simulink model "slexPowerWindowExample"  (R2014b)
settings: Solver=ode23  StartTime=0  StopTime=10  RelTol=1e-3
PreLoadFcn:
  | if ~exist('CV', 'var') & exist('slexPowerWindowContinuous','file')
  |    slexPowerWindowContinuous
  | end
libraries: slexPowerWindowSALib x8, slrtlib x2, slexPowerWindowDSPLib x2, slexPowerWindowPHYSLib x2, powerlib x1, vrlib x1
CloseFcn:
  | if exist('slexPowerWindowCloseFcn','file')
  |   slexPowerWindowCloseFcn
  | end
Description:
  | Main Power Window Model
settings Model: ModifiedByFormat=The MathWorks Inc.  Creator=The MathWorks Inc.  LastModifiedBy=The MathWorks Inc.
settings SolverCC: InsertRTBMode=Always
settings DataIOCC: SaveFormat=StructureWithTime  InspectSignalLogs=on  SignalLoggingName=sigsOut
settings OptimizationCC: ExpressionDepthLimit=2147483647
settings DebuggingCC: ArrayBoundsChecking=warning  UnderspecifiedInitializationDetection=Classic  MergeDetectMultiDrivingBlocksExec=none  SolverPrmCheckMsg=none  SigSpecEnsureSampleTimeMsg=none  ParameterPrecisionLossMsg=none  StateNameClashWarn=warning
settings ModelReferenceCC: ModelReferencePassRootInputsByReference=off
settings SimMechanicsCC: WarnOnRedundantConstraints=off

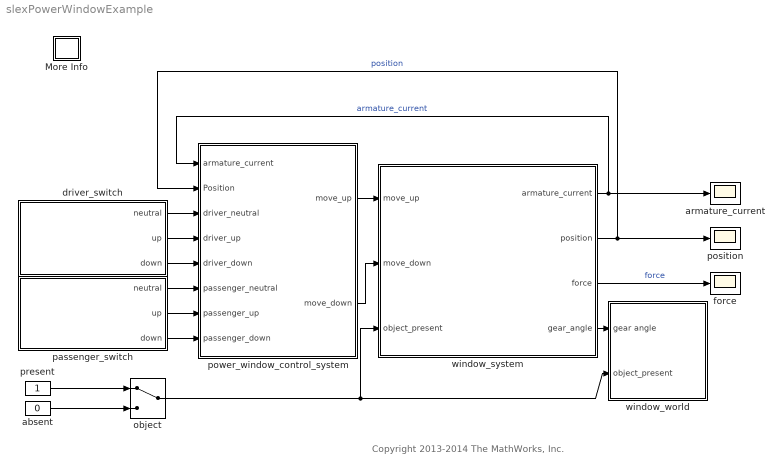
== system slexPowerWindowExample ==
  note: Copyright 2013-2014 The MathWorks, Inc.
  More Info : Subsystem
      settings: OpenFcn=showdemo('slexPowerWindowScript')
      mask Display: disp('?')
  absent : Constant  Value=0  OutDataTypeStr=boolean
  armature_current : Scope
      settings: YMin=-15  YMax=15  SaveName=ScopeData2
  driver_switch : Subsystem  Variant=on
  force : Scope
      settings: YMin=-175  YMax=75  SaveName=ScopeData4
  object : ManualSwitch
  passenger_switch : Subsystem  Variant=on
  position : Scope
      settings: TimeRange=10  YMin=-0.5  YMax=0.5
  power_window_control_system : Subsystem
  present : Constant  OutDataTypeStr=boolean
  window_system : Subsystem  Variant=on
  window_world : Subsystem  LoadFcn=|  Variant=on
      | if license('test','virtual_reality_toolbox') & exist('slexPowerWindowMechWindow.wrl','file')
      |      SL3DBlock = [gcs '/window_world/Simulink_3D_Animation View/VR Sink'];
      |      vrmfunc('FnOpen', get_param(SL3DBlock,'handle'));
      | end
  wires:
  passenger_switch/1(neutral) -> power_window_control_system/6(passenger_neutral)
  passenger_switch/2(up) -> power_window_control_system/7(passenger_up)
  passenger_switch/3(down) -> power_window_control_system/8(passenger_down)
  driver_switch/3(down) -> power_window_control_system/5(driver_down)
  driver_switch/2(up) -> power_window_control_system/4(driver_up)
  driver_switch/1(neutral) -> power_window_control_system/3(driver_neutral)
  power_window_control_system/1(move_up) -> window_system/1(move_up)
  power_window_control_system/2(move_down) -> window_system/2(move_down)
  window_system/1(armature_current) -> power_window_control_system/1(armature_current), armature_current/1  "armature_current"
  window_system/4(gear_angle) -> window_world/1(gear angle)
  window_system/3(force) -> force/1  "force"
  present/1 -> object/1
  absent/1 -> object/2
  window_system/2(position) -> power_window_control_system/2(Position), position/1  "position"
  object/1 -> window_system/3(object_present), window_world/2(object_present)

== system slexPowerWindowExample/More Info ==

== system slexPowerWindowExample/driver_switch ==
  Communication Protocol : Subsystem  VariantControl=V5
  Normal : slexPowerWindowSALib/switch  VariantControl=V1234
  neutral : Outport
  up : Outport  Port=2
  down : Outport  Port=3

== system slexPowerWindowExample/passenger_switch ==
  Communication Protocol : Subsystem  VariantControl=V5
  Normal : slexPowerWindowSALib/switch  VariantControl=V1234
  neutral : Outport
  up : Outport  Port=2
  down : Outport  Port=3

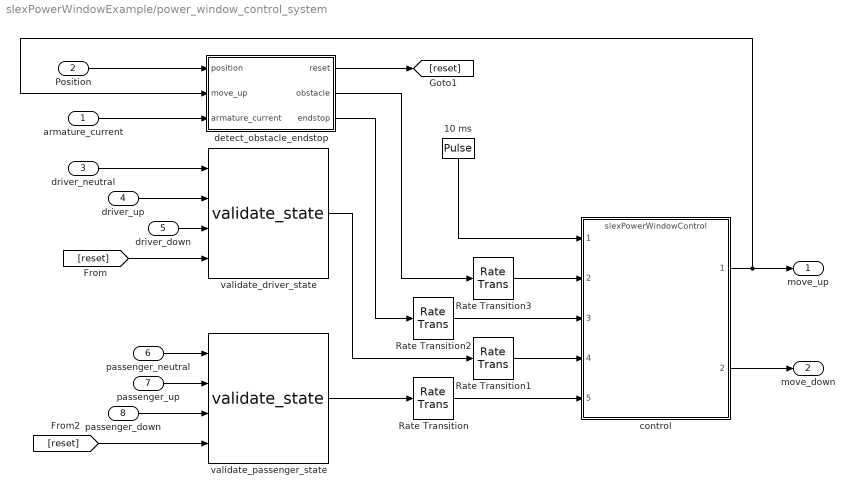
== system slexPowerWindowExample/power_window_control_system ==
  armature_current : Inport
  Position : Inport  Port=2
  driver_neutral : Inport  Port=3
  driver_up : Inport  Port=4
  driver_down : Inport  Port=5
  passenger_neutral : Inport  Port=6
  passenger_up : Inport  Port=7
  passenger_down : Inport  Port=8
  10 ms : DiscretePulseGenerator  SampleTime=10e-3
  Rate Transition{,1..3} (4 alike) : RateTransition
  "control " : ModelReference  ModelNameDialog=slexPowerWindowControl.slx  SimulationMode=Normal  ModelReferenceVersion=1.83  CopyOfModelName=slexPowerWindowControl.slx  DefaultDataLogging=on
  detect_obstacle_endstop : Subsystem  Variant=on
  validate_driver_state : slexPowerWindowSALib/validate_state
  validate_passenger_state : slexPowerWindowSALib/validate_state
  move_up : Outport
  move_down : Outport  Port=2
  wires:
  [reset] -> validate_driver_state/4
  driver_neutral/1 -> validate_driver_state/1
  driver_up/1 -> validate_driver_state/2
  driver_down/1 -> validate_driver_state/3
  detect_obstacle_endstop/1(reset) -> [reset]
  armature_current/1 -> detect_obstacle_endstop/3(armature_current)
  Position/1 -> detect_obstacle_endstop/1(position)
  "control "/1 -> move_up/1, detect_obstacle_endstop/2(move_up)
  "control "/2 -> move_down/1
  passenger_up/1 -> validate_passenger_state/2
  passenger_down/1 -> validate_passenger_state/3
  [reset] -> validate_passenger_state/4
  passenger_neutral/1 -> validate_passenger_state/1
  10 ms/1 -> "control "/1
  validate_passenger_state/1 -> Rate Transition/1
  validate_driver_state/1 -> Rate Transition1/1
  detect_obstacle_endstop/3(endstop) -> Rate Transition2/1
  detect_obstacle_endstop/2(obstacle) -> Rate Transition3/1
  Rate Transition/1 -> "control "/5
  Rate Transition1/1 -> "control "/4
  Rate Transition2/1 -> "control "/3
  Rate Transition3/1 -> "control "/2

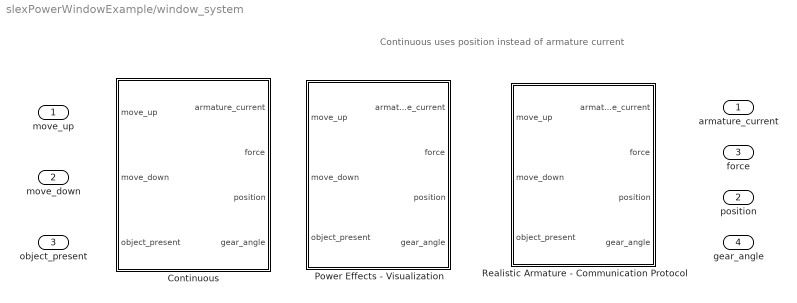
== system slexPowerWindowExample/window_system ==
  note: Continuous uses position instead of armature current
  move_up : Inport
  move_down : Inport  Port=2
  object_present : Inport  Port=3
  Continuous : Subsystem  VariantControl=V1
  Power Effects - Visualization : Subsystem  VariantControl=V23
  Realistic Armature - Communication Protocol : Subsystem  VariantControl=V45
  armature_current : Outport
  position : Outport  Port=2
  force : Outport  Port=3
  gear_angle : Outport  Port=4

== system slexPowerWindowExample/window_world ==
  gear angle : Inport
  object_present : Inport  Port=2
  No_View : Subsystem  VariantControl=V0
  Simulink_3D_Animation View : Subsystem  VariantControl=V12345

== system slexPowerWindowExample/driver_switch/Communication Protocol ==
  driver bit-unpacking1 : slrtlib/CAN/Utilities/CAN bit-unpacking   bitpatterns={ [0:0] [1:1] [2:2] }  dtypes={ 'boolean' 'boolean' 'boolean' }
  driver window control switch : slexPowerWindowDSPLib/driver window control switch
  neutral : Outport
  up : Outport  Port=2
  down : Outport  Port=3
  wires:
  driver window control switch/1 -> driver bit-unpacking1/1
  driver bit-unpacking1/3 -> down/1
  driver bit-unpacking1/1 -> neutral/1
  driver bit-unpacking1/2 -> up/1

== system slexPowerWindowExample/passenger_switch/Communication Protocol ==
  passenger bit-unpacking : slrtlib/CAN/Utilities/CAN bit-unpacking   bitpatterns={ [0:0] [1:1] [2:2] }  dtypes={ 'boolean' 'boolean' 'boolean' }
  passenger window control switch : slexPowerWindowDSPLib/passenger window control switch
  neutral : Outport
  up : Outport  Port=2
  down : Outport  Port=3
  wires:
  passenger bit-unpacking/2 -> up/1
  passenger bit-unpacking/1 -> neutral/1
  passenger bit-unpacking/3 -> down/1
  passenger window control switch/1 -> passenger bit-unpacking/1

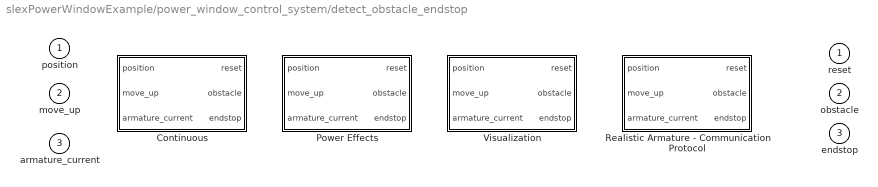
== system slexPowerWindowExample/power_window_control_system/detect_obstacle_endstop ==
  position : Inport
  move_up : Inport  Port=2
  armature_current : Inport  Port=3
  Continuous : Subsystem  VariantControl=V1
  Power Effects : Subsystem  VariantControl=V2
  Realistic Armature - Communication Protocol : Subsystem  VariantControl=V45
  Visualization : Subsystem  VariantControl=V3
  reset : Outport
  obstacle : Outport  Port=2
  endstop : Outport  Port=3

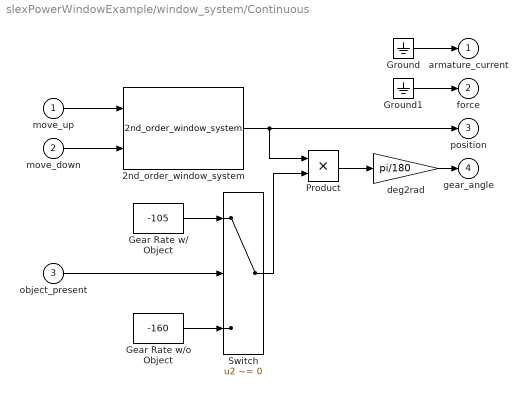
== system slexPowerWindowExample/window_system/Continuous ==
  move_up : Inport
  move_down : Inport  Port=2
  object_present : Inport  Port=3
  2nd_order_window_system : slexPowerWindowSALib/2nd_order_window_system
  Gear Rate w/ Object : Constant  Value=-105
      settings: AttributesFormatString=Units: deg/m
  Gear Rate w/o Object : Constant  Value=-160
      settings: AttributesFormatString=Units: deg/m
  Ground : Ground
  Ground1 : Ground
  Product : Product
  Switch : Switch  Criteria=u2 ~= 0
  deg2rad : Gain  Gain=pi/180
  armature_current : Outport
  force : Outport  Port=2
  position : Outport  Port=3
  gear_angle : Outport  Port=4
  wires:
  move_up/1 -> 2nd_order_window_system/1
  move_down/1 -> 2nd_order_window_system/2
  2nd_order_window_system/1 -> Product/1, position/1
  Ground/1 -> armature_current/1
  Ground1/1 -> force/1
  deg2rad/1 -> gear_angle/1
  object_present/1 -> Switch/2
  Product/1 -> deg2rad/1
  Switch/1 -> Product/2
  Gear Rate w/ Object/1 -> Switch/1
  Gear Rate w/o Object/1 -> Switch/3

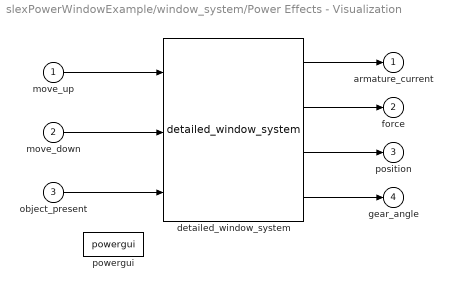
== system slexPowerWindowExample/window_system/Power Effects - Visualization ==
  move_up : Inport
  move_down : Inport  Port=2
  object_present : Inport  Port=3
  detailed_window_system : slexPowerWindowPHYSLib/detailed_window_system
  powergui : powerlib/powergui  SimulationMode=Continuous  SolverType=Tustin  SampleTime=50e-6  frequency=60  SPID=off  DisableSnubberDevices=off  DisableRonSwitches=off  DisableVfSwitches=off  SwTol=0  Interpol=off  DisplayEquations=off  Ts=0  methode=off  frequencyindice=0  Pbase=100e6  ErrMax=1e-4  Iterations=50  UnitsV=kV  UnitsW=MW  FunctionMessages=on  echomessages=off  HookPort=off  EnableUseOfTLC=off  x0status=blocks  RestoreLinks=warning  ResistiveCurrentMeasurement=off  Frange=[0:2:500]  Ylog=off  Xlog=on  ShowGrid=off  save=off  variable=ZData  structure=0  ZoomFFT=on  StartTime=0.0  cycles=1  DisplayStyle=1  fundamental=60  FreqAxis=off  MaxFrequency=1000  frequencyindicesteady=1  RmsSteady=1  display=off
  armature_current : Outport
  force : Outport  Port=2
  position : Outport  Port=3
  gear_angle : Outport  Port=4
  wires:
  detailed_window_system/1 -> armature_current/1
  detailed_window_system/2 -> force/1
  detailed_window_system/3 -> position/1
  detailed_window_system/4 -> gear_angle/1
  move_down/1 -> detailed_window_system/2
  move_up/1 -> detailed_window_system/1
  object_present/1 -> detailed_window_system/3

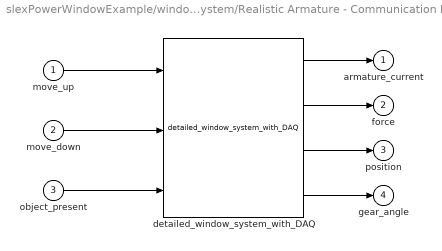
== system slexPowerWindowExample/window_system/Realistic Armature - Communication Protocol ==
  move_up : Inport
  move_down : Inport  Port=2
  object_present : Inport  Port=3
  detailed_window_system_with_DAQ : slexPowerWindowPHYSLib/detailed_window_system_with_DAQ  VariantControl=Variant3
  armature_current : Outport
  force : Outport  Port=2
  position : Outport  Port=3
  gear_angle : Outport  Port=4
  wires:
  detailed_window_system_with_DAQ/1 -> armature_current/1
  detailed_window_system_with_DAQ/2 -> force/1
  detailed_window_system_with_DAQ/3 -> position/1
  detailed_window_system_with_DAQ/4 -> gear_angle/1
  move_down/1 -> detailed_window_system_with_DAQ/2
  move_up/1 -> detailed_window_system_with_DAQ/1
  object_present/1 -> detailed_window_system_with_DAQ/3

== system slexPowerWindowExample/window_world/No_View ==
  gear angle : Inport
  object_present : Inport  Port=2
  Terminator : Terminator
  Terminator1 : Terminator
  wires:
  object_present/1 -> Terminator/1
  gear angle/1 -> Terminator1/1

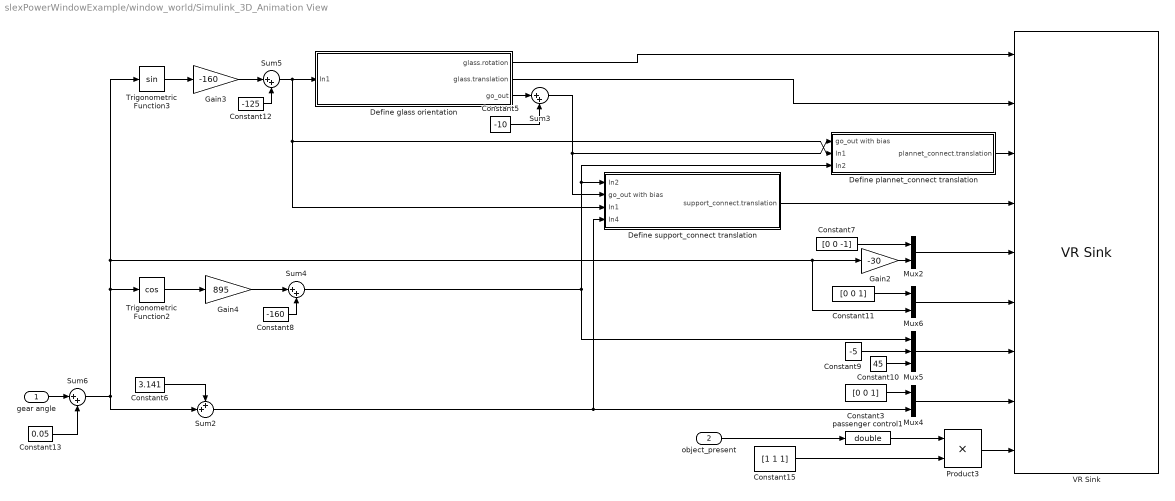
== system slexPowerWindowExample/window_world/Simulink_3D_Animation View ==
  gear angle : Inport
  object_present : Inport  Port=2
  Constant10 : Constant  Value=45
  Constant11 : Constant  Value=[0 0 1]
  Constant12 : Constant  Value=-125
  Constant13 : Constant  Value=0.05
  Constant15 : Constant  Value=[1 1 1]
  Constant3 : Constant  Value=[0 0 1]
  Constant5 : Constant  Value=-10
  Constant6 : Constant  Value=3.141
  Constant7 : Constant  Value=[0 0 -1]
  Constant8 : Constant  Value=-160
  Constant9 : Constant  Value=-5
  Define glass orientation : Subsystem
  Define plannet_connect translation : Subsystem
  Define support_connect translation : Subsystem
  Gain2 : Gain  Gain=-30  SaturateOnIntegerOverflow=on  OutDataTypeStr=Inherit: Same as input  ParamDataTypeStr=Inherit: Same as input
  Gain3 : Gain  Gain=-160  SaturateOnIntegerOverflow=on  OutDataTypeStr=Inherit: Same as input  ParamDataTypeStr=Inherit: Same as input
  Gain4 : Gain  Gain=895  SaturateOnIntegerOverflow=on  OutDataTypeStr=Inherit: Same as input  ParamDataTypeStr=Inherit: Same as input
  Mux2 : Mux  Inputs=2
  Mux4 : Mux  Inputs=2
  Mux5 : Mux  Inputs=3
  Mux6 : Mux  Inputs=2
  Product3 : Product  SaturateOnIntegerOverflow=on  InputSameDT=on  OutDataTypeStr=Inherit: Same as first input
  Sum2 : Sum  Inputs=++|  SaturateOnIntegerOverflow=on  InputSameDT=on  OutDataTypeStr=Inherit: Same as first input
  Sum{3..6} (4 alike) : Sum  Inputs=|++  SaturateOnIntegerOverflow=on  InputSameDT=on  OutDataTypeStr=Inherit: Same as first input
  Trigonometric Function2 : Trigonometry  Operator=cos
  Trigonometric Function3 : Trigonometry
  VR Sink : vrlib/VR Sink  InstantiateOnLoad=on  SampleTime=0.1  ViewEnable=on  RemoteChange=off  RemoteView=on  FieldsWritten=glass.rotation.4.1.1.double#glass.translation.3.1.1.double#plannet_connect.translation.3.1.1.double#support_connect.translation.3.1.1.double#worm.rotation.4.1.1.double#planetROT.rotation.4.1.1.double#support.translation.3.1.1.double#supportROT.rotation.4.1.1.double#balloon.scale.3.1.1.double  WorldFileName=slexPowerWindowMechWindow.wrl  WorldDescription=VR Power Window Model  AutoView=off  VideoDimensions=[]  AllowVariableSize=off  FigureProperties="{'Position', 'Name', 'Viewpoint', 'CameraBound', 'CameraDirection', 'CameraPosition', 'CameraUpVector', 'ZoomFactor', 'Antialiasing', 'Headlight', 'Lighting', 'NavPanel', 'StatusBar', 'ToolBar', 'Textures', 'Transparency', 'Triad', 'Wireframe', 'NavZones', 'NavMode', 'NavSpeed', 'CaptureFileFormat', 'CaptureFileName', 'Record2DCompressMethod', 'Record2DCompressQuality', 'Record2D', 'Record2DFileName', 'Record2DFPS'; [1.0000000000000000e+00   8.9000000000000000e+01   5.8400000000000000e+02   3.8400000000000000e+02], 'VR Power Window Model', 'Main View', 'on', [0.0000000000000000e+00   0.0000000000000000e+00  -1.0000000000000000e+00], [0.0000000000000000e+00   0.0000000000000000e+00   0.0000000000000000e+00], [0.0000000000000000e+00   1.0000000000000000e+00   0.0000000000000000e+00], [1.0000000000000000e+00], 'on', 'on', 'on', 'halfbar', 'on', 'on', 'on', 'on', 'none', 'off', 'off', 'examine', 'normal', 'tif', '%f_anim_%n.tif', 'auto', [7.5000000000000000e+01], 'off', '%f_anim_%n.avi', [1.5000000000000000e+01]}"
  passenger control1 : DataTypeConversion  OutDataTypeStr=double  SaturateOnIntegerOverflow=on  RndMeth=Zero
  wires:
  Mux2/1 -> VR Sink/5
  Mux6/1 -> VR Sink/6
  Mux5/1 -> VR Sink/7
  Define support_connect translation/1(support_connect.translation) -> VR Sink/4
  Product3/1 -> VR Sink/9
  Constant5/1 -> Sum3/2
  Constant7/1 -> Mux2/1
  Gain2/1 -> Mux2/2
  Gain3/1 -> Sum5/1
  Constant12/1 -> Sum5/2
  Constant11/1 -> Mux6/1
  Trigonometric Function3/1 -> Gain3/1
  Constant8/1 -> Sum4/2
  Gain4/1 -> Sum4/1
  Trigonometric Function2/1 -> Gain4/1
  Constant9/1 -> Mux5/2
  Constant10/1 -> Mux5/3
  Sum2/1 -> Mux4/2, Define support_connect translation/4(In4)
  Constant3/1 -> Mux4/1
  gear angle/1 -> Sum6/1
  passenger control1/1 -> Product3/1
  Constant13/1 -> Sum6/2
  Constant15/1 -> Product3/2
  object_present/1 -> passenger control1/1
  Define glass orientation/3(go_out) -> Sum3/1
  Sum6/1 -> Sum2/2, Trigonometric Function2/1, Trigonometric Function3/1, Gain2/1, Mux6/2
  Sum3/1 -> Define plannet_connect translation/1(go_out with bias), Define support_connect translation/2(go_out with bias)
  Sum5/1 -> Define plannet_connect translation/2(In1), Define support_connect translation/3(In1), Define glass orientation/1(In1)
  Sum4/1 -> Mux5/1, Define support_connect translation/1(In2), Define plannet_connect translation/3(In2)
  Constant6/1 -> Sum2/1
  Define glass orientation/1(glass.rotation) -> VR Sink/1
  Define glass orientation/2(glass.translation) -> VR Sink/2
  Define plannet_connect translation/1(plannet_connect.translation) -> VR Sink/3
  Mux4/1 -> VR Sink/8

== system slexPowerWindowExample/power_window_control_system/detect_obstacle_endstop/Continuous ==
  position : Inport
  move_up : Inport  Port=2
  armature_current : Inport  Port=3
  Terminator : Terminator
  verify_position : slexPowerWindowSALib/verify_position
  reset : Outport
  obstacle : Outport  Port=2
  endstop : Outport  Port=3
  wires:
  verify_position/1 -> reset/1
  armature_current/1 -> Terminator/1
  position/1 -> verify_position/1
  move_up/1 -> verify_position/2
  verify_position/2 -> obstacle/1
  verify_position/3 -> endstop/1

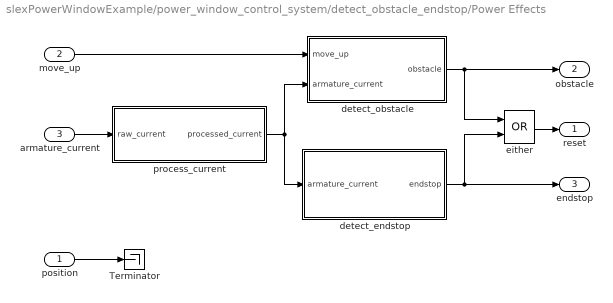
== system slexPowerWindowExample/power_window_control_system/detect_obstacle_endstop/Power Effects ==
  position : Inport
  move_up : Inport  Port=2
  armature_current : Inport  Port=3
  Terminator : Terminator
  detect_endstop : Subsystem
  detect_obstacle : Subsystem
  either : Logic  Operator=OR
  process_current : Subsystem
  reset : Outport
  obstacle : Outport  Port=2
  endstop : Outport  Port=3
  wires:
  process_current/1(processed_current) -> detect_endstop/1(armature_current), detect_obstacle/2(armature_current)
  move_up/1 -> detect_obstacle/1(move_up)
  either/1 -> reset/1
  detect_endstop/1(endstop) -> either/2, endstop/1
  detect_obstacle/1(obstacle) -> obstacle/1, either/1
  armature_current/1 -> process_current/1(raw_current)
  position/1 -> Terminator/1

== system slexPowerWindowExample/power_window_control_system/detect_obstacle_endstop/Realistic Armature - Communication Protocol ==
  position : Inport
  move_up : Inport  Port=2
  armature_current : Inport  Port=3
  Terminator : Terminator
  fp_verify_current : slexPowerWindowSALib/fp_verify_current
  reset : Outport
  obstacle : Outport  Port=2
  endstop : Outport  Port=3
  wires:
  fp_verify_current/1 -> reset/1
  armature_current/1 -> fp_verify_current/2
  position/1 -> Terminator/1
  fp_verify_current/2 -> obstacle/1
  fp_verify_current/3 -> endstop/1
  move_up/1 -> fp_verify_current/1

== system slexPowerWindowExample/power_window_control_system/detect_obstacle_endstop/Visualization ==
  position : Inport
  move_up : Inport  Port=2
  armature_current : Inport  Port=3
  Terminator : Terminator
  verify_current : slexPowerWindowSALib/verify_current
  reset : Outport
  obstacle : Outport  Port=2
  endstop : Outport  Port=3
  wires:
  verify_current/1 -> reset/1
  armature_current/1 -> verify_current/2
  position/1 -> Terminator/1
  move_up/1 -> verify_current/1
  verify_current/2 -> obstacle/1
  verify_current/3 -> endstop/1

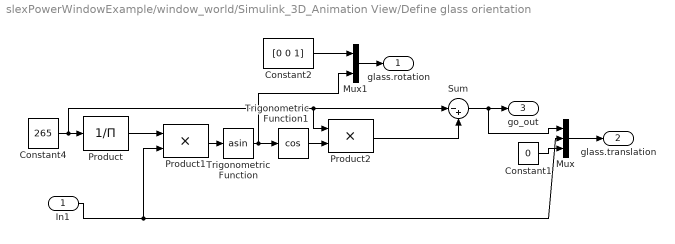
== system slexPowerWindowExample/window_world/Simulink_3D_Animation View/Define glass orientation ==
  In1 : Inport
  Constant1 : Constant  Value=0
  Constant2 : Constant  Value=[0 0 1]
  Constant4 : Constant  Value=265
  Mux : Mux  Inputs=3
  Mux1 : Mux  Inputs=2
  Product : Product  Inputs=/  SaturateOnIntegerOverflow=on  InputSameDT=on  OutDataTypeStr=Inherit: Same as first input
  Product1 : Product  SaturateOnIntegerOverflow=on  InputSameDT=on  OutDataTypeStr=Inherit: Same as first input
  Product2 : Product  SaturateOnIntegerOverflow=on  InputSameDT=on  OutDataTypeStr=Inherit: Same as first input
  Sum : Sum  Inputs=|-+  SaturateOnIntegerOverflow=on  InputSameDT=on  OutDataTypeStr=Inherit: Same as first input
  Trigonometric Function : Trigonometry  Operator=asin
  Trigonometric Function1 : Trigonometry  Operator=cos
  glass.rotation : Outport
  glass.translation : Outport  Port=2
  go_out : Outport  Port=3
  wires:
  Mux/1 -> glass.translation/1
  Mux1/1 -> glass.rotation/1
  In1/1 -> Product1/2, Mux/2
  Constant1/1 -> Mux/3
  Constant2/1 -> Mux1/1
  Constant4/1 -> Product/1, Product2/1, Sum/1
  Product/1 -> Product1/1
  Product1/1 -> Trigonometric Function/1
  Trigonometric Function/1 -> Trigonometric Function1/1, Mux1/2
  Trigonometric Function1/1 -> Product2/2
  Product2/1 -> Sum/2
  Sum/1 -> go_out/1, Mux/1

== system slexPowerWindowExample/window_world/Simulink_3D_Animation View/Define plannet_connect translation ==
  go_out with bias : Inport
  In1 : Inport  Port=2
  In2 : Inport  Port=3
  Gain1 : Gain  Gain=0.265  SaturateOnIntegerOverflow=on  OutDataTypeStr=Inherit: Same as input  ParamDataTypeStr=Inherit: Same as input
  Mux3 : Mux  Inputs=3
  plannet_connect.translation : Outport
  wires:
  Mux3/1 -> plannet_connect.translation/1
  In2/1 -> Gain1/1
  In1/1 -> Mux3/2
  go_out with bias/1 -> Mux3/1
  Gain1/1 -> Mux3/3

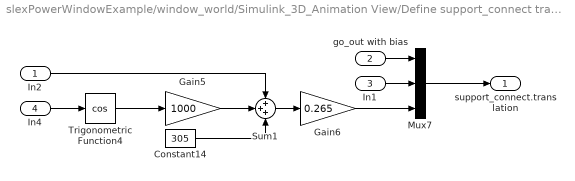
== system slexPowerWindowExample/window_world/Simulink_3D_Animation View/Define support_connect translation ==
  In2 : Inport
  go_out with bias : Inport  Port=2
  In1 : Inport  Port=3
  In4 : Inport  Port=4
  Constant14 : Constant  Value=305
  Gain5 : Gain  Gain=1000  SaturateOnIntegerOverflow=on  OutDataTypeStr=Inherit: Same as input  ParamDataTypeStr=Inherit: Same as input
  Gain6 : Gain  Gain=0.265  SaturateOnIntegerOverflow=on  OutDataTypeStr=Inherit: Same as input  ParamDataTypeStr=Inherit: Same as input
  Mux7 : Mux  Inputs=3
  Sum1 : Sum  Inputs=+++  SaturateOnIntegerOverflow=on  InputSameDT=on  OutDataTypeStr=Inherit: Same as first input
  Trigonometric Function4 : Trigonometry  Operator=cos
  support_connect.translation : Outport
  wires:
  Mux7/1 -> support_connect.translation/1
  In4/1 -> Trigonometric Function4/1
  In2/1 -> Sum1/1
  In1/1 -> Mux7/2
  go_out with bias/1 -> Mux7/1
  Trigonometric Function4/1 -> Gain5/1
  Gain5/1 -> Sum1/2
  Sum1/1 -> Gain6/1
  Gain6/1 -> Mux7/3
  Constant14/1 -> Sum1/3

== system slexPowerWindowExample/power_window_control_system/detect_obstacle_endstop/Power Effects/detect_endstop ==
  armature_current : Inport
  Constant6 : Constant  Value=15
  current_limit : RelationalOperator  Operator=>  InputSameDT=on
  endstop : Outport
  wires:
  Constant6/1 -> current_limit/2
  armature_current/1 -> current_limit/1
  current_limit/1 -> endstop/1

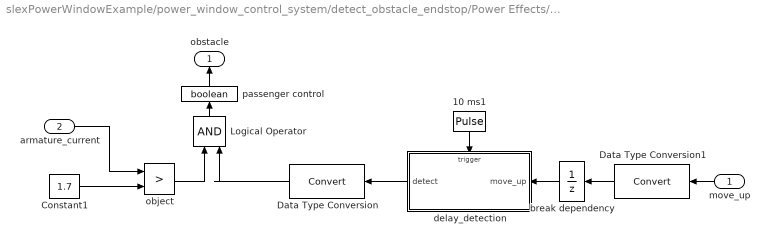
== system slexPowerWindowExample/power_window_control_system/detect_obstacle_endstop/Power Effects/detect_obstacle ==
  move_up : Inport
  armature_current : Inport  Port=2
  10 ms1 : DiscretePulseGenerator  SampleTime=10e-3
  Constant1 : Constant  Value=1.7
  Data Type Conversion : DataTypeConversion
  Data Type Conversion1 : DataTypeConversion
  Logical Operator : Logic  IconShape=distinctive  AllPortsSameDT=off  OutDataTypeStr=boolean
  break dependency : UnitDelay  SampleTime=0.01
  delay_detection : Stateflow chart  TreatAsAtomicUnit=on
  object : RelationalOperator  Operator=>  InputSameDT=on
  passenger control : DataTypeConversion  OutDataTypeStr=boolean  SaturateOnIntegerOverflow=on  RndMeth=Zero
  obstacle : Outport
  wires:
  Constant1/1 -> object/2
  object/1 -> Logical Operator/1
  delay_detection/1(" detect") -> Data Type Conversion/1
  armature_current/1 -> object/1
  move_up/1 -> Data Type Conversion1/1
  Logical Operator/1 -> passenger control/1
  10 ms1/1 -> delay_detection/Trigger
  break dependency/1 -> delay_detection/1(move_up)
  passenger control/1 -> obstacle/1
  Data Type Conversion1/1 -> break dependency/1
  Data Type Conversion/1 -> Logical Operator/2

== system slexPowerWindowExample/power_window_control_system/detect_obstacle_endstop/Power Effects/process_current ==
  raw_current : Inport
  Abs : Abs  SaturateOnIntegerOverflow=on
  processed_current : Outport
  wires:
  Abs/1 -> processed_current/1
  raw_current/1 -> Abs/1

== stateflow chart slexPowerWindowExample/power_window_control_system/detect_obstacle_endstop/Power Effects/detect_obstacle/delay_detection ==
  settings: executeAtInitialization=1
  state off
  state hold
  state detect
  (default) -> off
  off -> hold : [move_up]
  detect -> off : [~move_up]
  hold -> off [order 2] : [~move_up]
  hold -> detect [order 1] : [after(100,ticks)]
  data: detect output unknown; move_up input boolean
  events: ticks input EITHER_EDGE_EVENT
